simulink model "nn_fuel_control_4_20_1"  (R2021a)
settings: Solver=ode15s  StartTime=0.0  StopTime=T  MaxStep=.01  RelTol=1e-3
undefined symbols (not defined in the file): AF_sensor_tol, fault_time, fuel_inj_tol, kappa_tol, MAF_sensor_tol, pump_tol, tau_ww_tol
libraries: neural x86
(part 2 of 4)

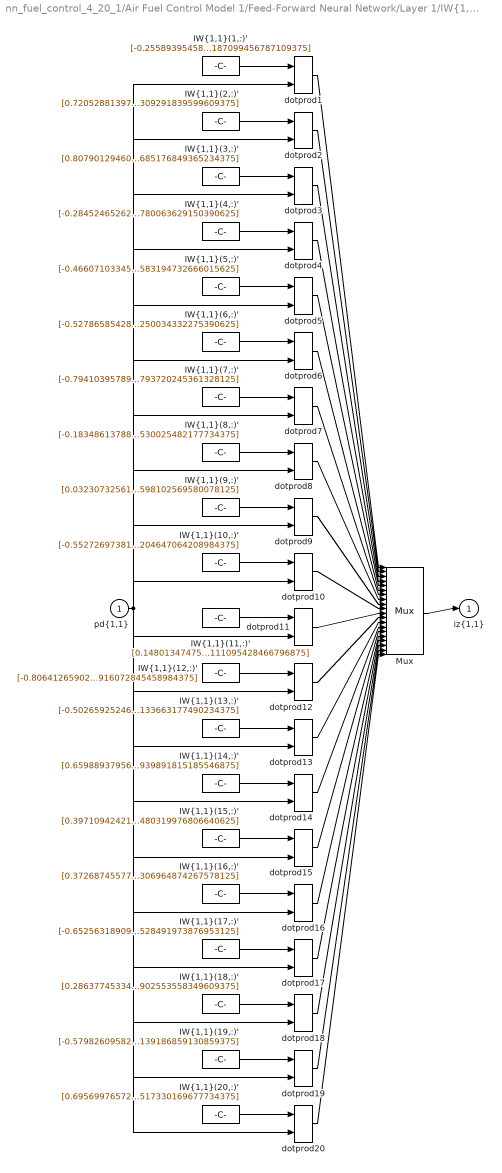
== system nn_fuel_control_4_20_1/Air Fuel Control Model 1/Feed-Forward Neural Network/Layer 1/IW{1,1} ==
  "pd{1,1}" : Inport  PortDimensions=4
      mask Display: e = 0.06;c1 = [120 230 180]/255;c2 = ([120 230 180]+0)/(256+128);c3 = ([120 230 180]+128)/(256+128);patch([0 1 1 0],[0 0 1 1],c1);patch([0 1 1 1-e 1-e 0+e],[0 0 1 1-e 0+e 0+e],c2);patch([0 0 1 1-e 0+e 0+e],[0 1 1 1-e 1-e 0+e],c3);plot([0 1 1 0 0],[0 0 1 1 0]);
  "IW{1,1}(1,:)'" : Constant  Value=[-0.255893954581917271173807648665388114750385284423828125;-0.050180613703053662810749102618501638062298297882080078125;-0.411204029772260393205129958005272783339023590087890625;-0.05416988303420254557973834153017378412187099456787109375]
      mask Display: e = 0.06;c1 = [120 150 230]/255;c2 = ([120 150 230]+0)/383;c3 = ([120 150 230]+128)/383;patch([0 1 1 0],[0 0 1 1],c1);patch([0 1 1 1-e 1-e 0+e],[0 0 1 1-e 0+e 0+e],c2);patch([0 0 1 1-e 0+e 0+e],[0 1 1 1-e 1-e 0+e],c3);plot([0 1 1 0 0],[0 0 1 1 0]);disp('Weights');
  "IW{1,1}(10,:)'" : Constant  Value=[-0.55272697381055768683921769479638896882534027099609375;-0.651499269241095912974515158566646277904510498046875;0.63947614252412832147598464871407486498355865478515625;-0.590736262891938590513518647640012204647064208984375]
      mask Display: e = 0.06;c1 = [120 150 230]/255;c2 = ([120 150 230]+0)/383;c3 = ([120 150 230]+128)/383;patch([0 1 1 0],[0 0 1 1],c1);patch([0 1 1 1-e 1-e 0+e],[0 0 1 1-e 0+e 0+e],c2);patch([0 0 1 1-e 0+e 0+e],[0 1 1 1-e 1-e 0+e],c3);plot([0 1 1 0 0],[0 0 1 1 0]);disp('Weights');
  "IW{1,1}(11,:)'" : Constant  Value=[0.1480134747547011409007922111413790844380855560302734375;0.6684648726112827343825983916758559644222259521484375;0.062198838454765502381516029117847210727632045745849609375;-0.60427407435323476914135198967414908111095428466796875]
      mask Display: e = 0.06;c1 = [120 150 230]/255;c2 = ([120 150 230]+0)/383;c3 = ([120 150 230]+128)/383;patch([0 1 1 0],[0 0 1 1],c1);patch([0 1 1 1-e 1-e 0+e],[0 0 1 1-e 0+e 0+e],c2);patch([0 0 1 1-e 0+e 0+e],[0 1 1 1-e 1-e 0+e],c3);plot([0 1 1 0 0],[0 0 1 1 0]);disp('Weights');
  "IW{1,1}(12,:)'" : Constant  Value=[-0.8064126590285745077579804274137131869792938232421875;-0.1946243266823513007324208956561051309108734130859375;0.05077726277785125919006503636410343460738658905029296875;0.71413696176898555645351507337181828916072845458984375]
      mask Display: e = 0.06;c1 = [120 150 230]/255;c2 = ([120 150 230]+0)/383;c3 = ([120 150 230]+128)/383;patch([0 1 1 0],[0 0 1 1],c1);patch([0 1 1 1-e 1-e 0+e],[0 0 1 1-e 0+e 0+e],c2);patch([0 0 1 1-e 0+e 0+e],[0 1 1 1-e 1-e 0+e],c3);plot([0 1 1 0 0],[0 0 1 1 0]);disp('Weights');
  "IW{1,1}(13,:)'" : Constant  Value=[-0.5026592524653068494444596581161022186279296875;-0.8442232439786565567629850193043239414691925048828125;-0.4600549917996483717530509238713420927524566650390625;-0.538643370776307417457928750081919133663177490234375]
      mask Display: e = 0.06;c1 = [120 150 230]/255;c2 = ([120 150 230]+0)/383;c3 = ([120 150 230]+128)/383;patch([0 1 1 0],[0 0 1 1],c1);patch([0 1 1 1-e 1-e 0+e],[0 0 1 1-e 0+e 0+e],c2);patch([0 0 1 1-e 0+e 0+e],[0 1 1 1-e 1-e 0+e],c3);plot([0 1 1 0 0],[0 0 1 1 0]);disp('Weights');
  "IW{1,1}(14,:)'" : Constant  Value=[0.6598893795696885167245682168868370354175567626953125;-0.66306349623711835494788147116196341812610626220703125;-0.016209493408949893211712378615629859268665313720703125;0.7971581335749486907360505938413552939891815185546875]
      mask Display: e = 0.06;c1 = [120 150 230]/255;c2 = ([120 150 230]+0)/383;c3 = ([120 150 230]+128)/383;patch([0 1 1 0],[0 0 1 1],c1);patch([0 1 1 1-e 1-e 0+e],[0 0 1 1-e 0+e 0+e],c2);patch([0 0 1 1-e 0+e 0+e],[0 1 1 1-e 1-e 0+e],c3);plot([0 1 1 0 0],[0 0 1 1 0]);disp('Weights');
  "IW{1,1}(15,:)'" : Constant  Value=[0.397109424219522555432604349334724247455596923828125;-0.97950665478874388014673968427814543247222900390625;-0.532533438767095912425020287628285586833953857421875;0.594249136505285324716396644362248480319976806640625]
      mask Display: e = 0.06;c1 = [120 150 230]/255;c2 = ([120 150 230]+0)/383;c3 = ([120 150 230]+128)/383;patch([0 1 1 0],[0 0 1 1],c1);patch([0 1 1 1-e 1-e 0+e],[0 0 1 1-e 0+e 0+e],c2);patch([0 0 1 1-e 0+e 0+e],[0 1 1 1-e 1-e 0+e],c3);plot([0 1 1 0 0],[0 0 1 1 0]);disp('Weights');
  "IW{1,1}(16,:)'" : Constant  Value=[0.372687455772187814506679615078610368072986602783203125;-0.90807611825004019845408720357227139174938201904296875;-0.457367237946180560381748136933310888707637786865234375;0.55645598307857035980106275019352324306964874267578125]
      mask Display: e = 0.06;c1 = [120 150 230]/255;c2 = ([120 150 230]+0)/383;c3 = ([120 150 230]+128)/383;patch([0 1 1 0],[0 0 1 1],c1);patch([0 1 1 1-e 1-e 0+e],[0 0 1 1-e 0+e 0+e],c2);patch([0 0 1 1-e 0+e 0+e],[0 1 1 1-e 1-e 0+e],c3);plot([0 1 1 0 0],[0 0 1 1 0]);disp('Weights');
  "IW{1,1}(17,:)'" : Constant  Value=[-0.6525631890917888977554639495792798697948455810546875;0.30110178388549169170573804876767098903656005859375;0.1303703819094477467377402035708655603229999542236328125;0.897007452078188993738194767502136528491973876953125]
      mask Display: e = 0.06;c1 = [120 150 230]/255;c2 = ([120 150 230]+0)/383;c3 = ([120 150 230]+128)/383;patch([0 1 1 0],[0 0 1 1],c1);patch([0 1 1 1-e 1-e 0+e],[0 0 1 1-e 0+e 0+e],c2);patch([0 0 1 1-e 0+e 0+e],[0 1 1 1-e 1-e 0+e],c3);plot([0 1 1 0 0],[0 0 1 1 0]);disp('Weights');
  "IW{1,1}(18,:)'" : Constant  Value=[0.286377453348653665532452805564389564096927642822265625;0.50923809025101751668529459493583999574184417724609375;-0.1177085687787508827550908563353004865348339080810546875;0.214421817752911803012239033705554902553558349609375]
      mask Display: e = 0.06;c1 = [120 150 230]/255;c2 = ([120 150 230]+0)/383;c3 = ([120 150 230]+128)/383;patch([0 1 1 0],[0 0 1 1],c1);patch([0 1 1 1-e 1-e 0+e],[0 0 1 1-e 0+e 0+e],c2);patch([0 0 1 1-e 0+e 0+e],[0 1 1 1-e 1-e 0+e],c3);plot([0 1 1 0 0],[0 0 1 1 0]);disp('Weights');
  "IW{1,1}(19,:)'" : Constant  Value=[-0.57982609582202027098674079752527177333831787109375;-0.563291776334291949268617827328853309154510498046875;0.100587291224137675982319706236012279987335205078125;0.1910173290938883550182936232886277139186859130859375]
      mask Display: e = 0.06;c1 = [120 150 230]/255;c2 = ([120 150 230]+0)/383;c3 = ([120 150 230]+128)/383;patch([0 1 1 0],[0 0 1 1],c1);patch([0 1 1 1-e 1-e 0+e],[0 0 1 1-e 0+e 0+e],c2);patch([0 0 1 1-e 0+e 0+e],[0 1 1 1-e 1-e 0+e],c3);plot([0 1 1 0 0],[0 0 1 1 0]);disp('Weights');
  "IW{1,1}(2,:)'" : Constant  Value=[0.72052881397894197323950038480688817799091339111328125;-0.1079570095728306367011128941157949157059192657470703125;0.280125365935717851595398997233132831752300262451171875;-0.31323344257810281643372718463069759309291839599609375]
      mask Display: e = 0.06;c1 = [120 150 230]/255;c2 = ([120 150 230]+0)/383;c3 = ([120 150 230]+128)/383;patch([0 1 1 0],[0 0 1 1],c1);patch([0 1 1 1-e 1-e 0+e],[0 0 1 1-e 0+e 0+e],c2);patch([0 0 1 1-e 0+e 0+e],[0 1 1 1-e 1-e 0+e],c3);plot([0 1 1 0 0],[0 0 1 1 0]);disp('Weights');
  "IW{1,1}(20,:)'" : Constant  Value=[0.69569976572952452187337257782928645610809326171875;-0.158886500019682130879772330445121042430400848388671875;1.0467247081747499404258405775181017816066741943359375;-0.786786319988487914400820955052040517330169677734375]
      mask Display: e = 0.06;c1 = [120 150 230]/255;c2 = ([120 150 230]+0)/383;c3 = ([120 150 230]+128)/383;patch([0 1 1 0],[0 0 1 1],c1);patch([0 1 1 1-e 1-e 0+e],[0 0 1 1-e 0+e 0+e],c2);patch([0 0 1 1-e 0+e 0+e],[0 1 1 1-e 1-e 0+e],c3);plot([0 1 1 0 0],[0 0 1 1 0]);disp('Weights');
  "IW{1,1}(3,:)'" : Constant  Value=[0.80790129460351567391995786238112486898899078369140625;0.60020113472108682639571952677215449512004852294921875;-0.743655296177256008860467773047275841236114501953125;-0.1015119663675712879946644306983216665685176849365234375]
      mask Display: e = 0.06;c1 = [120 150 230]/255;c2 = ([120 150 230]+0)/383;c3 = ([120 150 230]+128)/383;patch([0 1 1 0],[0 0 1 1],c1);patch([0 1 1 1-e 1-e 0+e],[0 0 1 1-e 0+e 0+e],c2);patch([0 0 1 1-e 0+e 0+e],[0 1 1 1-e 1-e 0+e],c3);plot([0 1 1 0 0],[0 0 1 1 0]);disp('Weights');
  "IW{1,1}(4,:)'" : Constant  Value=[-0.28452465262175674620692689131828956305980682373046875;-0.1455400286438181256531976259793736971914768218994140625;0.2090543561159994012665919171922723762691020965576171875;0.3143679152500846729623162900679744780063629150390625]
      mask Display: e = 0.06;c1 = [120 150 230]/255;c2 = ([120 150 230]+0)/383;c3 = ([120 150 230]+128)/383;patch([0 1 1 0],[0 0 1 1],c1);patch([0 1 1 1-e 1-e 0+e],[0 0 1 1-e 0+e 0+e],c2);patch([0 0 1 1-e 0+e 0+e],[0 1 1 1-e 1-e 0+e],c3);plot([0 1 1 0 0],[0 0 1 1 0]);disp('Weights');
  "IW{1,1}(5,:)'" : Constant  Value=[-0.46607103345306055697250258162966929376125335693359375;0.4045752847885430991681232626433484256267547607421875;-0.2487346108752874485059436437950353138148784637451171875;-0.8540124870413221547238435960025526583194732666015625]
      mask Display: e = 0.06;c1 = [120 150 230]/255;c2 = ([120 150 230]+0)/383;c3 = ([120 150 230]+128)/383;patch([0 1 1 0],[0 0 1 1],c1);patch([0 1 1 1-e 1-e 0+e],[0 0 1 1-e 0+e 0+e],c2);patch([0 0 1 1-e 0+e 0+e],[0 1 1 1-e 1-e 0+e],c3);plot([0 1 1 0 0],[0 0 1 1 0]);disp('Weights');
  "IW{1,1}(6,:)'" : Constant  Value=[-0.52786585428759724702985067779081873595714569091796875;0.56258148622816828154924451155238784849643707275390625;0.1597122724516217562307218713613110594451427459716796875;-0.56017202948027000619646287304931320250034332275390625]
      mask Display: e = 0.06;c1 = [120 150 230]/255;c2 = ([120 150 230]+0)/383;c3 = ([120 150 230]+128)/383;patch([0 1 1 0],[0 0 1 1],c1);patch([0 1 1 1-e 1-e 0+e],[0 0 1 1-e 0+e 0+e],c2);patch([0 0 1 1-e 0+e 0+e],[0 1 1 1-e 1-e 0+e],c3);plot([0 1 1 0 0],[0 0 1 1 0]);disp('Weights');
  "IW{1,1}(7,:)'" : Constant  Value=[-0.7941039578996564873847319177002646028995513916015625;0.402454842875472562635508211315027438104152679443359375;-1.1760264490640590651082675321958959102630615234375;0.4049690339423961393805484476615674793720245361328125]
      mask Display: e = 0.06;c1 = [120 150 230]/255;c2 = ([120 150 230]+0)/383;c3 = ([120 150 230]+128)/383;patch([0 1 1 0],[0 0 1 1],c1);patch([0 1 1 1-e 1-e 0+e],[0 0 1 1-e 0+e 0+e],c2);patch([0 0 1 1-e 0+e 0+e],[0 1 1 1-e 1-e 0+e],c3);plot([0 1 1 0 0],[0 0 1 1 0]);disp('Weights');
  "IW{1,1}(8,:)'" : Constant  Value=[-0.1834861378839762746650876579224132001399993896484375;-0.2696005694128247309748758198111318051815032958984375;0.0449899432481253302995582998846657574176788330078125;0.40879506644844099128022207878530025482177734375]
      mask Display: e = 0.06;c1 = [120 150 230]/255;c2 = ([120 150 230]+0)/383;c3 = ([120 150 230]+128)/383;patch([0 1 1 0],[0 0 1 1],c1);patch([0 1 1 1-e 1-e 0+e],[0 0 1 1-e 0+e 0+e],c2);patch([0 0 1 1-e 0+e 0+e],[0 1 1 1-e 1-e 0+e],c3);plot([0 1 1 0 0],[0 0 1 1 0]);disp('Weights');
  "IW{1,1}(9,:)'" : Constant  Value=[0.0323073256130863573076794637017883360385894775390625;0.3668530899902517905530885400366969406604766845703125;-0.620161838295766099093953016563318669795989990234375;-0.9815621933458509307257600084994919598102569580078125]
      mask Display: e = 0.06;c1 = [120 150 230]/255;c2 = ([120 150 230]+0)/383;c3 = ([120 150 230]+128)/383;patch([0 1 1 0],[0 0 1 1],c1);patch([0 1 1 1-e 1-e 0+e],[0 0 1 1-e 0+e 0+e],c2);patch([0 0 1 1-e 0+e 0+e],[0 1 1 1-e 1-e 0+e],c3);plot([0 1 1 0 0],[0 0 1 1 0]);disp('Weights');
  Mux : Mux  Inputs=20
      mask Display: e = 0.06;c1 = [120 150 230]/255;c2 = ([120 150 230]+0)/383;c3 = ([120 150 230]+128)/383;patch([0 1 1 0],[0 0 1 1],c1);patch([0 1 1 1-e 1-e 0+e],[0 0 1 1-e 0+e 0+e],c2);patch([0 0 1 1-e 0+e 0+e],[0 1 1 1-e 1-e 0+e],c3);plot([0 1 1 0 0],[0 0 1 1 0]);disp('Mux');
  dotprod{1..20} (20 alike) : neural/Weight Functions/dotprod
  "iz{1,1}" : Outport
      mask Display: e = 0.06;c1 = [120 230 180]/255;c2 = ([120 230 180]+0)/(256+128);c3 = ([120 230 180]+128)/(256+128);patch([0 1 1 0],[0 0 1 1],c1);patch([0 1 1 1-e 1-e 0+e],[0 0 1 1-e 0+e 0+e],c2);patch([0 0 1 1-e 0+e 0+e],[0 1 1 1-e 1-e 0+e],c3);plot([0 1 1 0 0],[0 0 1 1 0]);
  wires:
  "IW{1,1}(1,:)'"/1 -> dotprod1/1
  "pd{1,1}"/1 -> dotprod1/2, dotprod2/2, dotprod3/2, dotprod4/2, dotprod5/2, dotprod6/2, dotprod7/2, dotprod8/2, dotprod9/2, dotprod10/2, dotprod11/2, dotprod12/2, dotprod13/2, dotprod14/2, dotprod15/2, dotprod16/2, dotprod17/2, dotprod18/2, dotprod19/2, dotprod20/2
  dotprod1/1 -> Mux/1
  "IW{1,1}(2,:)'"/1 -> dotprod2/1
  dotprod2/1 -> Mux/2
  "IW{1,1}(3,:)'"/1 -> dotprod3/1
  dotprod3/1 -> Mux/3
  "IW{1,1}(4,:)'"/1 -> dotprod4/1
  dotprod4/1 -> Mux/4
  "IW{1,1}(5,:)'"/1 -> dotprod5/1
  dotprod5/1 -> Mux/5
  "IW{1,1}(6,:)'"/1 -> dotprod6/1
  dotprod6/1 -> Mux/6
  "IW{1,1}(7,:)'"/1 -> dotprod7/1
  dotprod7/1 -> Mux/7
  "IW{1,1}(8,:)'"/1 -> dotprod8/1
  dotprod8/1 -> Mux/8
  "IW{1,1}(9,:)'"/1 -> dotprod9/1
  dotprod9/1 -> Mux/9
  "IW{1,1}(10,:)'"/1 -> dotprod10/1
  dotprod10/1 -> Mux/10
  "IW{1,1}(11,:)'"/1 -> dotprod11/1
  dotprod11/1 -> Mux/11
  "IW{1,1}(12,:)'"/1 -> dotprod12/1
  dotprod12/1 -> Mux/12
  "IW{1,1}(13,:)'"/1 -> dotprod13/1
  dotprod13/1 -> Mux/13
  "IW{1,1}(14,:)'"/1 -> dotprod14/1
  dotprod14/1 -> Mux/14
  "IW{1,1}(15,:)'"/1 -> dotprod15/1
  dotprod15/1 -> Mux/15
  "IW{1,1}(16,:)'"/1 -> dotprod16/1
  dotprod16/1 -> Mux/16
  "IW{1,1}(17,:)'"/1 -> dotprod17/1
  dotprod17/1 -> Mux/17
  "IW{1,1}(18,:)'"/1 -> dotprod18/1
  dotprod18/1 -> Mux/18
  "IW{1,1}(19,:)'"/1 -> dotprod19/1
  dotprod19/1 -> Mux/19
  "IW{1,1}(20,:)'"/1 -> dotprod20/1
  dotprod20/1 -> Mux/20
  Mux/1 -> "iz{1,1}"/1

== system nn_fuel_control_4_20_1/Air Fuel Control Model 1/Feed-Forward Neural Network/Layer 2/Delays 1 ==
  "p{2}" : Inport  PortDimensions=20
      mask Display: e = 0.06;c1 = [120 230 180]/255;c2 = ([120 230 180]+0)/(256+128);c3 = ([120 230 180]+128)/(256+128);patch([0 1 1 0],[0 0 1 1],c1);patch([0 1 1 1-e 1-e 0+e],[0 0 1 1-e 0+e 0+e],c2);patch([0 0 1 1-e 0+e 0+e],[0 1 1 1-e 1-e 0+e],c3);plot([0 1 1 0 0],[0 0 1 1 0]);
  mux : Mux  Inputs=1
      mask Display: e = 0.06;c1 = [120 150 230]/255;c2 = ([120 150 230]+0)/383;c3 = ([120 150 230]+128)/383;patch([0 1 1 0],[0 0 1 1],c1);patch([0 1 1 1-e 1-e 0+e],[0 0 1 1-e 0+e 0+e],c2);patch([0 0 1 1-e 0+e 0+e],[0 1 1 1-e 1-e 0+e],c3);plot([0 1 1 0 0],[0 0 1 1 0]);disp('Mux')
  "pd{2,1}" : Outport
      mask Display: e = 0.06;c1 = [120 230 180]/255;c2 = ([120 230 180]+0)/(256+128);c3 = ([120 230 180]+128)/(256+128);patch([0 1 1 0],[0 0 1 1],c1);patch([0 1 1 1-e 1-e 0+e],[0 0 1 1-e 0+e 0+e],c2);patch([0 0 1 1-e 0+e 0+e],[0 1 1 1-e 1-e 0+e],c3);plot([0 1 1 0 0],[0 0 1 1 0]);
  wires:
  "p{2}"/1 -> mux/1
  mux/1 -> "pd{2,1}"/1

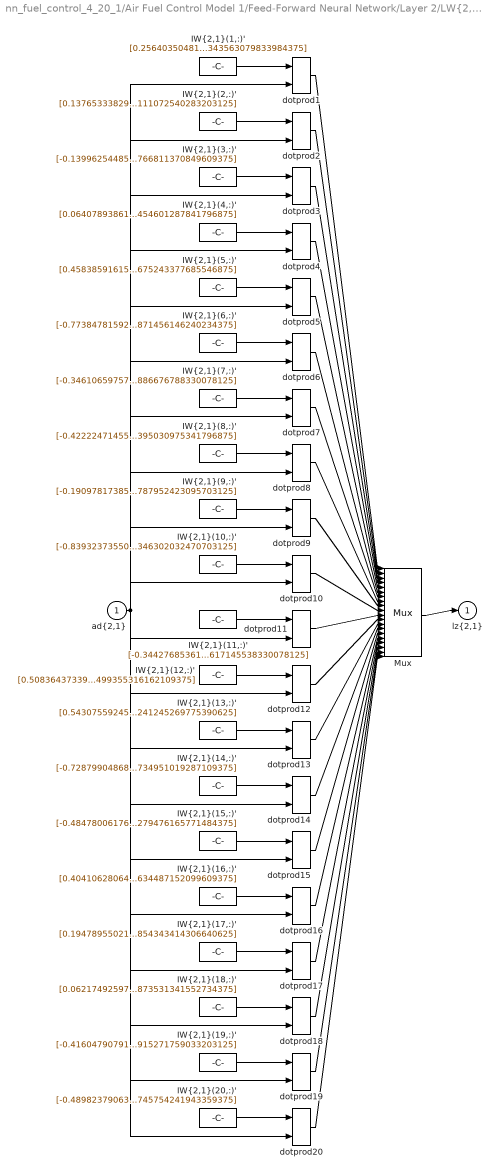
== system nn_fuel_control_4_20_1/Air Fuel Control Model 1/Feed-Forward Neural Network/Layer 2/LW{2,1} ==
  "ad{2,1}" : Inport  PortDimensions=20
      mask Display: e = 0.06;c1 = [120 230 180]/255;c2 = ([120 230 180]+0)/(256+128);c3 = ([120 230 180]+128)/(256+128);patch([0 1 1 0],[0 0 1 1],c1);patch([0 1 1 1-e 1-e 0+e],[0 0 1 1-e 0+e 0+e],c2);patch([0 0 1 1-e 0+e 0+e],[0 1 1 1-e 1-e 0+e],c3);plot([0 1 1 0 0],[0 0 1 1 0]);
  "IW{2,1}(1,:)'" : Constant  Value=[0.256403504819027683314658361268811859190464019775390625;0.55699273716688690871734479514998383820056915283203125;-0.10243484263037373749316572002499015070497989654541015625;0.61017359243633340071255588554777204990386962890625;-0.49168853908283549625224395640543662011623382568359375;-0.445185796413017254025135116535238921642303466796875;0.66658292791435036495073518381104804575443267822265625;0.74941831651127532865075409063138067722320556640625;0.348045444215012711453027804964222013950347900390625;0.86509340571704573807920723993447609245777130126953125;0.74428775142764858063770816443138755857944488525390625;-0.6684261822986099499388501499197445809841156005859375;0.821552287158203053962779449648223817348480224609375;0.06921567489521453231393621763345436193048954010009765625;0.69405408543870894533256432623602449893951416015625;-0.08884209416376896706335486442185356281697750091552734375;0.1065002363070592095173338975655497051775455474853515625;0.9502109393119704261465585659607313573360443115234375;0.3213179247461728227364119447884149849414825439453125;-0.48618430376372800960638187461881898343563079833984375]
      mask Display: e = 0.06;c1 = [120 150 230]/255;c2 = ([120 150 230]+0)/383;c3 = ([120 150 230]+128)/383;patch([0 1 1 0],[0 0 1 1],c1);patch([0 1 1 1-e 1-e 0+e],[0 0 1 1-e 0+e 0+e],c2);patch([0 0 1 1-e 0+e 0+e],[0 1 1 1-e 1-e 0+e],c3);plot([0 1 1 0 0],[0 0 1 1 0]);disp('weights');
  "IW{2,1}(10,:)'" : Constant  Value=[-0.839323735500342227311421083868481218814849853515625;-0.1027802378071994426900204189223586581647396087646484375;-0.7806964202693096321894472566782496869564056396484375;0.680681515772560086219300501397810876369476318359375;-0.51100504457678008751742027016007341444492340087890625;-0.51150485750802621165433947680867277085781097412109375;-0.1924599703979477938187159224980860017240047454833984375;-0.3642331759206876018453158394549973309040069580078125;0.4202409374541262732094537568627856671810150146484375;-0.64692134435889148136311632697470486164093017578125;-0.49688718155034805601388825380126945674419403076171875;0.5581295053278108042604799265973269939422607421875;-0.4857655414840549301658256808877922594547271728515625;-0.41702184565919953040946666078525595366954803466796875;-0.3202437589281850183198230297421105206012725830078125;-0.9406677162011334303315379656851291656494140625;0.7897233817597302252266899813548661768436431884765625;-0.70530703875142897185668289239401929080486297607421875;-0.197104048309090007506938491133041679859161376953125;-0.9954045937389335296785475293290801346302032470703125]
      mask Display: e = 0.06;c1 = [120 150 230]/255;c2 = ([120 150 230]+0)/383;c3 = ([120 150 230]+128)/383;patch([0 1 1 0],[0 0 1 1],c1);patch([0 1 1 1-e 1-e 0+e],[0 0 1 1-e 0+e 0+e],c2);patch([0 0 1 1-e 0+e 0+e],[0 1 1 1-e 1-e 0+e],c3);plot([0 1 1 0 0],[0 0 1 1 0]);disp('weights');
  "IW{2,1}(11,:)'" : Constant  Value=[-0.3442768536160334402751459492719732224941253662109375;-0.126645193186832150100684657445526681840419769287109375;-0.25582239816656604514122363980277441442012786865234375;-0.475188837819449261257176431172410957515239715576171875;-0.380699988172073233716474760512937791645526885986328125;0.6681082596167755571769930611480958759784698486328125;0.61680611870214019365477042811107821762561798095703125;-0.3842982728840949047111053005210123956203460693359375;0.092199959895641558915713176247663795948028564453125;0.646735751844751849404246968333609402179718017578125;-0.3566726201985510602554541037534363567829132080078125;0.862487777138273514765387517400085926055908203125;0.3401193911093225441533149933093227446079254150390625;-0.88438663542802509187623627440189011394977569580078125;-0.2883601808382836306776653145789168775081634521484375;1.13845020905304039615657529793679714202880859375;-0.98259045851291926254589270683936774730682373046875;0.3131654024901433519545435046893544495105743408203125;-0.40667411652741325411852812976576387882232666015625;0.88431093975587338196220343888853676617145538330078125]
      mask Display: e = 0.06;c1 = [120 150 230]/255;c2 = ([120 150 230]+0)/383;c3 = ([120 150 230]+128)/383;patch([0 1 1 0],[0 0 1 1],c1);patch([0 1 1 1-e 1-e 0+e],[0 0 1 1-e 0+e 0+e],c2);patch([0 0 1 1-e 0+e 0+e],[0 1 1 1-e 1-e 0+e],c3);plot([0 1 1 0 0],[0 0 1 1 0]);disp('weights');
  "IW{2,1}(12,:)'" : Constant  Value=[0.5083643733909475326271376616205088794231414794921875;0.6979322964989373989652676755213178694248199462890625;0.92178415717860884281975586418411694467067718505859375;-0.39033104832621534630021642442443408071994781494140625;-0.383678218211015054084356279417988844215869903564453125;-0.61391769395999717939815809586434625089168548583984375;-0.591094668264378952926563215442001819610595703125;-0.312979327589984368529485436738468706607818603515625;-0.0842029111634989835266651425627060234546661376953125;-0.8006509914526864779560355600551702082157135009765625;-0.10037107631365442539372878627546015195548534393310546875;0.551034974300382174305923399515450000762939453125;0.7040581567920323191600573409232310950756072998046875;0.059419260238086461789475123396186972968280315399169921875;0.483832787080651360867022958700545132160186767578125;-0.6947366657908133902310510165989398956298828125;0.188227171095658951660567481667385436594486236572265625;-0.24625857672740936177291359854280017316341400146484375;0.0379784065678607785088161108433268964290618896484375;-0.1936138778400245674671253937049186788499355316162109375]
      mask Display: e = 0.06;c1 = [120 150 230]/255;c2 = ([120 150 230]+0)/383;c3 = ([120 150 230]+128)/383;patch([0 1 1 0],[0 0 1 1],c1);patch([0 1 1 1-e 1-e 0+e],[0 0 1 1-e 0+e 0+e],c2);patch([0 0 1 1-e 0+e 0+e],[0 1 1 1-e 1-e 0+e],c3);plot([0 1 1 0 0],[0 0 1 1 0]);disp('weights');
  "IW{2,1}(13,:)'" : Constant  Value=[0.54307559245790348878557551870471797883510589599609375;0.75271368477932398821650394893367774784564971923828125;-0.1275235670257674203131870172001072205603122711181640625;-0.58684458116446325259829563947278074920177459716796875;0.9795271839011350234471819931059144437313079833984375;0.115565273299358672876024911602144129574298858642578125;0.11335394344267306354634428089411812834441661834716796875;0.358539371416803920311622277949936687946319580078125;-0.0126515875916339837203850038349628448486328125;-0.260894828747942231217393782571889460086822509765625;0.1574081397651138358728672983488650061190128326416015625;0.1420118999546165217129356506120529957115650177001953125;0.5099030275380067589452437459840439260005950927734375;-0.81828653190900879632607711755554191768169403076171875;-0.1545897804274993792006398507510311901569366455078125;0.675439808810708530728561527212150394916534423828125;-0.127791243383908181829866634870995767414569854736328125;0.98852637578982560651041922028525732457637786865234375;0.0986064542185760561920915279188193380832672119140625;0.01154229721346903582424037182363463216461241245269775390625]
      mask Display: e = 0.06;c1 = [120 150 230]/255;c2 = ([120 150 230]+0)/383;c3 = ([120 150 230]+128)/383;patch([0 1 1 0],[0 0 1 1],c1);patch([0 1 1 1-e 1-e 0+e],[0 0 1 1-e 0+e 0+e],c2);patch([0 0 1 1-e 0+e 0+e],[0 1 1 1-e 1-e 0+e],c3);plot([0 1 1 0 0],[0 0 1 1 0]);disp('weights');
  "IW{2,1}(14,:)'" : Constant  Value=[-0.728799048689657613664394375518895685672760009765625;-0.296529345416541800783960525222937576472759246826171875;-0.7972119443543326244849822614924050867557525634765625;-1.0118923326638957771450577638461254537105560302734375;-0.5272267009729585396371476235799491405487060546875;-0.8855868557823221021152448884095065295696258544921875;0.5121663467363941624199696889263577759265899658203125;0.2545828879630407381995382820605300366878509521484375;0.6292814383810225731252785408287309110164642333984375;-0.929475350504611608215554952039383351802825927734375;0.069808995965472020461817237446666695177555084228515625;0.7352931823411916756327855182462371885776519775390625;-0.7827631248789221896089429719722829759120941162109375;-0.537355068723539108788145313155837357044219970703125;0.4990633751586894817364736809395253658294677734375;0.10586567362169052586295947548933327198028564453125;0.7861825800106121420185445458628237247467041015625;-0.8456802487706689408497595650260336697101593017578125;-0.015314959104377745546798905706964433193206787109375;-0.2971057125480276450701921930885873734951019287109375]
      mask Display: e = 0.06;c1 = [120 150 230]/255;c2 = ([120 150 230]+0)/383;c3 = ([120 150 230]+128)/383;patch([0 1 1 0],[0 0 1 1],c1);patch([0 1 1 1-e 1-e 0+e],[0 0 1 1-e 0+e 0+e],c2);patch([0 0 1 1-e 0+e 0+e],[0 1 1 1-e 1-e 0+e],c3);plot([0 1 1 0 0],[0 0 1 1 0]);disp('weights');
  "IW{2,1}(15,:)'" : Constant  Value=[-0.484780061765159142606052000701311044394969940185546875;-0.415234292406290117494194191749556921422481536865234375;-1.0346574979893914392192755258292891085147857666015625;-0.402016275094312536264595792090403847396373748779296875;-0.138088078526567181736339762210263870656490325927734375;0.87346766333678382832061970475479029119014739990234375;0.441802139086038103688025557858054526150226593017578125;-0.1309872596360344143562315366580151021480560302734375;-0.610204389748495668044370177085511386394500732421875;-0.03839265832583131643485074846466886810958385467529296875;0.249243117002509839696955395993427373468875885009765625;0.11801074905021964600582151661001262255012989044189453125;-0.2659363890055583823368579032830893993377685546875;-0.71930459889416187291288906635600142180919647216796875;-0.075520266869505636719850372173823416233062744140625;0.06868026364486297385969493234370020218193531036376953125;-0.89298865365537405391904712814721278846263885498046875;-0.215387890558910999327935087421792559325695037841796875;-0.2384945521682781954808660884737037122249603271484375;-0.62116688404883591001492959549068473279476165771484375]
      mask Display: e = 0.06;c1 = [120 150 230]/255;c2 = ([120 150 230]+0)/383;c3 = ([120 150 230]+128)/383;patch([0 1 1 0],[0 0 1 1],c1);patch([0 1 1 1-e 1-e 0+e],[0 0 1 1-e 0+e 0+e],c2);patch([0 0 1 1-e 0+e 0+e],[0 1 1 1-e 1-e 0+e],c3);plot([0 1 1 0 0],[0 0 1 1 0]);disp('weights');
  "IW{2,1}(16,:)'" : Constant  Value=[0.404106280640281256832935241618542931973934173583984375;0.70242360718233898264628578544943593442440032958984375;0.1641145711031210263630697454573237337172031402587890625;-0.247221087020352836560732612269930541515350341796875;0.05562678511628217636886262198459007777273654937744140625;-0.0072461926376732911647682300326778204180300235748291015625;0.1324024557175408622899936972316936589777469635009765625;-0.92978342018724191575529403053224086761474609375;0.56556497776320835413343957043252885341644287109375;0.3397230627633225363837254917598329484462738037109375;0.29431922470979732242568616129574365913867950439453125;0.51626009844002884729974311994737945497035980224609375;-0.6489613631160897622152106123394332826137542724609375;-0.24239263777640218666675764325191266834735870361328125;-0.5586844817010707675564162855152972042560577392578125;0.0290138265195338147794945626856133458204567432403564453125;0.6115143731481691435902803277713246643543243408203125;0.1748207830102221638224335720224189572036266326904296875;0.4941049018132852577167568597360514104366302490234375;0.33386371882758003604152463594800792634487152099609375]
      mask Display: e = 0.06;c1 = [120 150 230]/255;c2 = ([120 150 230]+0)/383;c3 = ([120 150 230]+128)/383;patch([0 1 1 0],[0 0 1 1],c1);patch([0 1 1 1-e 1-e 0+e],[0 0 1 1-e 0+e 0+e],c2);patch([0 0 1 1-e 0+e 0+e],[0 1 1 1-e 1-e 0+e],c3);plot([0 1 1 0 0],[0 0 1 1 0]);disp('weights');
  "IW{2,1}(17,:)'" : Constant  Value=[0.1947895502174626092273257427223143167793750762939453125;-0.52361898938939310799156601206050254404544830322265625;-0.10622093506646522464986759359817369841039180755615234375;-0.7466049808737535986580269309342838823795318603515625;0.427384088335486078680247601369046606123447418212890625;1.4693398718208683373376288727740757167339324951171875;-1.3104810676142888414830167675972916185855865478515625;0.4855049744317463389364775139256380498409271240234375;0.88199212165116680495202672318555414676666259765625;-0.60955399776535756917184016856481321156024932861328125;-0.54285148849283759719952513478347100317478179931640625;-0.70516678840002133821229790555662475526332855224609375;-0.41511492758453183427036492503248155117034912109375;0.6704157094871272537517370437853969633579254150390625;0.839123341803627909030183218419551849365234375;0.63222268412543380922130609178566373884677886962890625;-0.50732264518261949159949608656461350619792938232421875;-0.74154304207597621090286565959104336798191070556640625;-0.8111671411077410187573377697844989597797393798828125;-0.428285368422044288028160963222035206854343414306640625]
      mask Display: e = 0.06;c1 = [120 150 230]/255;c2 = ([120 150 230]+0)/383;c3 = ([120 150 230]+128)/383;patch([0 1 1 0],[0 0 1 1],c1);patch([0 1 1 1-e 1-e 0+e],[0 0 1 1-e 0+e 0+e],c2);patch([0 0 1 1-e 0+e 0+e],[0 1 1 1-e 1-e 0+e],c3);plot([0 1 1 0 0],[0 0 1 1 0]);disp('weights');
  "IW{2,1}(18,:)'" : Constant  Value=[0.06217492597023745182216458715629414655268192291259765625;-0.81824560730074236136744048053515143692493438720703125;-0.89641287430782690126562783916597254574298858642578125;-0.18391094474156732818670434426167048513889312744140625;0.9844616979050770932957448167144320905208587646484375;0.65484074414303805600212626814027316868305206298828125;-0.7925667457472191923528725965297780930995941162109375;0.0673400334330274130678617439116351306438446044921875;-0.083604201131516564515777645283378660678863525390625;0.58893929866951510998518415362923406064510345458984375;-0.94534449182464685978999341386952437460422515869140625;0.457648829261737388751640764894546009600162506103515625;0.1025857773266978245629843513597734272480010986328125;0.54381759553698583165015634222072549164295196533203125;0.5443058289233437818666061502881348133087158203125;-1.036147741921205511772541285608895123004913330078125;-0.24802282339544390321606215366045944392681121826171875;-0.9227639004882857154399289356661029160022735595703125;0.010338230956161709173102281056344509124755859375;-0.22463957916662502523053035474731586873531341552734375]
      mask Display: e = 0.06;c1 = [120 150 230]/255;c2 = ([120 150 230]+0)/383;c3 = ([120 150 230]+128)/383;patch([0 1 1 0],[0 0 1 1],c1);patch([0 1 1 1-e 1-e 0+e],[0 0 1 1-e 0+e 0+e],c2);patch([0 0 1 1-e 0+e 0+e],[0 1 1 1-e 1-e 0+e],c3);plot([0 1 1 0 0],[0 0 1 1 0]);disp('weights');
  "IW{2,1}(19,:)'" : Constant  Value=[-0.416047907917482195916392129220184870064258575439453125;0.309121326860066714115049535394064150750637054443359375;-0.0851180957864090814712909605077584274113178253173828125;0.339056785143795114123577150166966021060943603515625;-0.3096899454485384506341461019474081695079803466796875;-0.027548179279832142596351474139737547375261783599853515625;0.5216670052960143966203077070531435310840606689453125;-0.9988357428048779684814917345647700130939483642578125;-0.0344484434883864931720154345384798943996429443359375;-0.13242871890093044218161821845569647848606109619140625;0.522090219246575060196846607141196727752685546875;0.59382139028936331559549444136791862547397613525390625;-0.472735042050936637991753741516731679439544677734375;-0.74187595298605690796733824754483066499233245849609375;0.9082521364400701902042101210099644958972930908203125;0.551414488237109257084966884576715528964996337890625;0.2127486436982679307572396965042571537196636199951171875;0.91331207772785572007734344879281707108020782470703125;-0.8915657199296169732605221724952571094036102294921875;0.304700671032038183927426189256948418915271759033203125]
      mask Display: e = 0.06;c1 = [120 150 230]/255;c2 = ([120 150 230]+0)/383;c3 = ([120 150 230]+128)/383;patch([0 1 1 0],[0 0 1 1],c1);patch([0 1 1 1-e 1-e 0+e],[0 0 1 1-e 0+e 0+e],c2);patch([0 0 1 1-e 0+e 0+e],[0 1 1 1-e 1-e 0+e],c3);plot([0 1 1 0 0],[0 0 1 1 0]);disp('weights');
  "IW{2,1}(2,:)'" : Constant  Value=[0.137653338293227733846180171894957311451435089111328125;-0.460904548992435214582741309641278348863124847412109375;-0.290558282766146314113342441487475298345088958740234375;-0.63113207125823567178457551563042216002941131591796875;-0.517856009400533334741112412302754819393157958984375;-0.522612663993072157353481088648550212383270263671875;-1.14371085022362262151318645919673144817352294921875;-0.296969721859859259183167523588053882122039794921875;0.024219358823902581434595049358904361724853515625;0.247160225307312242382096201254171319305896759033203125;0.46439009629174032856013809578143991529941558837890625;0.053387629679267745164139569169492460787296295166015625;-0.1041289206064270889129375063930638134479522705078125;-0.00838366847669662351716368675624835304915904998779296875;-0.0691640104665527388760892790742218494415283203125;0.259218969043773894700422033565700985491275787353515625;0.197015094634830856268337129222345538437366485595703125;-0.171531257694670757896204804637818597257137298583984375;0.3180435006853030710516350154648534953594207763671875;0.00376749716591924521669199066309374757111072540283203125]
      mask Display: e = 0.06;c1 = [120 150 230]/255;c2 = ([120 150 230]+0)/383;c3 = ([120 150 230]+128)/383;patch([0 1 1 0],[0 0 1 1],c1);patch([0 1 1 1-e 1-e 0+e],[0 0 1 1-e 0+e 0+e],c2);patch([0 0 1 1-e 0+e 0+e],[0 1 1 1-e 1-e 0+e],c3);plot([0 1 1 0 0],[0 0 1 1 0]);disp('weights');
  "IW{2,1}(20,:)'" : Constant  Value=[-0.48982379063714720501820920617319643497467041015625;-0.1565414567378254073748422570133698172867298126220703125;1.0092678630572751163896327852853573858737945556640625;0.04997173210835093026815911798621527850627899169921875;-0.2079386696337817141966297640465199947357177734375;-0.321525828659411760934716539850342087447643280029296875;0.89409571631389106460829907518927939236164093017578125;0.5543458800608702663481608396978117525577545166015625;-0.49306510763555611021047297981567680835723876953125;0.27814303195336009810745281356503255665302276611328125;-0.81464293081563654563836962552159093320369720458984375;-0.35123732988197675641828254811116494238376617431640625;0.559540544336689205096035948372446000576019287109375;0.74652085046993865713460536426282487809658050537109375;0.28824650081486868913316357065923511981964111328125;-0.6182866746032604776672769730794243514537811279296875;-1.0877338496879047635701454055379144847393035888671875;-0.104371293272435661236841042409650981426239013671875;-0.913504009541565853425026944023557007312774658203125;-0.07584107192232168725976038103908649645745754241943359375]
      mask Display: e = 0.06;c1 = [120 150 230]/255;c2 = ([120 150 230]+0)/383;c3 = ([120 150 230]+128)/383;patch([0 1 1 0],[0 0 1 1],c1);patch([0 1 1 1-e 1-e 0+e],[0 0 1 1-e 0+e 0+e],c2);patch([0 0 1 1-e 0+e 0+e],[0 1 1 1-e 1-e 0+e],c3);plot([0 1 1 0 0],[0 0 1 1 0]);disp('weights');
  "IW{2,1}(3,:)'" : Constant  Value=[-0.13996254485875747608503161245607770979404449462890625;0.40060507371922027264332655249745585024356842041015625;-0.56815400850477704164376291373628191649913787841796875;-0.36553702608923399619555993922404013574123382568359375;-0.2482509998169468434792150901557761244475841522216796875;0.87407339206503975592710276032448746263980865478515625;0.893528192848337621256860074936412274837493896484375;0.632635861991303727336344309151172637939453125;0.869699939278778533235936265555210411548614501953125;0.98773112363063086949210855891578830778598785400390625;0.85399909375677662826120695171994157135486602783203125;-0.32594369818186275100657667280756868422031402587890625;0.4629603075816663970698527919012121856212615966796875;0.04308516642885058811618392837772262282669544219970703125;-0.231801523593062608341597297112457454204559326171875;-1.1623640803209145389018885907717049121856689453125;-0.88408872473551369797206689327140338718891143798828125;-0.8663309035618642628406860239920206367969512939453125;0.765185547700010459948316565714776515960693359375;-0.58307506602012215690677976454026065766811370849609375]
      mask Display: e = 0.06;c1 = [120 150 230]/255;c2 = ([120 150 230]+0)/383;c3 = ([120 150 230]+128)/383;patch([0 1 1 0],[0 0 1 1],c1);patch([0 1 1 1-e 1-e 0+e],[0 0 1 1-e 0+e 0+e],c2);patch([0 0 1 1-e 0+e 0+e],[0 1 1 1-e 1-e 0+e],c3);plot([0 1 1 0 0],[0 0 1 1 0]);disp('weights');
  "IW{2,1}(4,:)'" : Constant  Value=[0.064078938617030456459389142764848656952381134033203125;-0.067040192438827472809492746819159947335720062255859375;-0.028600678525859624112825940756010822951793670654296875;-0.452359910631902006894478063259157352149486541748046875;0.4009867174625458829950730432756245136260986328125;-0.239822770647339866822989051797776482999324798583984375;-0.470685619005303923501060126000083982944488525390625;-0.4068062304188486688616421815822832286357879638671875;0.9372201712705725551444402299239300191402435302734375;-0.99400142862411744459905094117857515811920166015625;-0.75301749780288673719041980803012847900390625;-0.234045308748025815415161332566640339791774749755859375;0.373406685408792071712014148943126201629638671875;-1.0597994395055365668412150625954382121562957763671875;0.314222984186316889321233247756026685237884521484375;-0.2078736406071655107297146969358436763286590576171875;-0.418901817343616700295427790479152463376522064208984375;-0.008801912503494602191267404123209416866302490234375;0.7107362770348044644919127676985226571559906005859375;0.7168103316080010056765559056657366454601287841796875]
      mask Display: e = 0.06;c1 = [120 150 230]/255;c2 = ([120 150 230]+0)/383;c3 = ([120 150 230]+128)/383;patch([0 1 1 0],[0 0 1 1],c1);patch([0 1 1 1-e 1-e 0+e],[0 0 1 1-e 0+e 0+e],c2);patch([0 0 1 1-e 0+e 0+e],[0 1 1 1-e 1-e 0+e],c3);plot([0 1 1 0 0],[0 0 1 1 0]);disp('weights');
  "IW{2,1}(5,:)'" : Constant  Value=[0.458385916159752326848320080898702144622802734375;0.84813204407613385082953527671634219586849212646484375;0.94650514098018889708185952258645556867122650146484375;0.74594759247516162492530611416441388428211212158203125;-0.104407762306979901012482514488510787487030029296875;0.1186644642958175899227768468335852958261966705322265625;1.1320098295769753793393874730099923908710479736328125;-0.179500407650915239088362795882858335971832275390625;0.771881138648502496124592653359286487102508544921875;-0.548635947097185994181245405343361198902130126953125;-0.6746199449777219303570063857478089630603790283203125;-0.360703913511002005609640264083282090723514556884765625;-0.597605875234097805304145367699675261974334716796875;-0.2568202039282214688142857994535006582736968994140625;0.5941759809159934402345015769242309033870697021484375;-0.039514724787864351218669156651230878196656703948974609375;0.229408580836399644820033927317126654088497161865234375;0.3342008973025247797750125755555927753448486328125;0.9800633193214773886126067736768163740634918212890625;0.5721963713908120308104798823478631675243377685546875]
      mask Display: e = 0.06;c1 = [120 150 230]/255;c2 = ([120 150 230]+0)/383;c3 = ([120 150 230]+128)/383;patch([0 1 1 0],[0 0 1 1],c1);patch([0 1 1 1-e 1-e 0+e],[0 0 1 1-e 0+e 0+e],c2);patch([0 0 1 1-e 0+e 0+e],[0 1 1 1-e 1-e 0+e],c3);plot([0 1 1 0 0],[0 0 1 1 0]);disp('weights');
  "IW{2,1}(6,:)'" : Constant  Value=[-0.77384781592172646735861007982748560607433319091796875;0.59108358077430744881297641768469475209712982177734375;-0.03728241009351639101421227451282902620732784271240234375;-0.97709174729592696007074437147821299731731414794921875;-0.7147538303215750232766367844305932521820068359375;-0.7829717176517638765886886176303960382938385009765625;-0.294662176883997595222552945415372960269451141357421875;-0.944338143760384607361402231617830693721771240234375;-0.17518116218259738303686390281654894351959228515625;0.51402311101222941669419697063858620822429656982421875;-0.99002176729454915982131524287979118525981903076171875;0.59043122934621827813117533878539688885211944580078125;-0.22370698215694329036296039703302085399627685546875;-1.056867006809679931933487750939093530178070068359375;0.4898055941529031453995912670507095754146575927734375;-0.6821680952663047303730081694084219634532928466796875;0.11879445532585231060096475630416534841060638427734375;-0.9976352361648259670090510553563944995403289794921875;-0.25460723909267901632347275153733789920806884765625;0.71721151247017311813891637939377687871456146240234375]
      mask Display: e = 0.06;c1 = [120 150 230]/255;c2 = ([120 150 230]+0)/383;c3 = ([120 150 230]+128)/383;patch([0 1 1 0],[0 0 1 1],c1);patch([0 1 1 1-e 1-e 0+e],[0 0 1 1-e 0+e 0+e],c2);patch([0 0 1 1-e 0+e 0+e],[0 1 1 1-e 1-e 0+e],c3);plot([0 1 1 0 0],[0 0 1 1 0]);disp('weights');
  "IW{2,1}(7,:)'" : Constant  Value=[-0.346106597572619578695451991734444163739681243896484375;0.399965489278604924283655464023468084633350372314453125;0.05447508061110746535593563066868227906525135040283203125;-0.87040339931752341851023402341525070369243621826171875;0.73883982147536653162234188130241818726062774658203125;0.427854113066676700061208293845993466675281524658203125;0.01403070065209728600752470129009452648460865020751953125;0.4861792379995455437580176294432021677494049072265625;0.9094214428940137207035832034307532012462615966796875;-0.03207414214986463452117249062212067656219005584716796875;-0.348223319994564739499054439875180833041667938232421875;0.269391913218515022254706536841695196926593780517578125;0.29729876555941192606269396492280066013336181640625;-0.3376447225389271888928988119005225598812103271484375;0.05065007115898811917986677144654095172882080078125;0.192316247203768775353438513775472529232501983642578125;0.02751917507898900272511610864967224188148975372314453125;0.54788988685930639643828499174560420215129852294921875;-0.0493641951991126148868715972639620304107666015625;-0.4195018892299196000550409735296852886676788330078125]
      mask Display: e = 0.06;c1 = [120 150 230]/255;c2 = ([120 150 230]+0)/383;c3 = ([120 150 230]+128)/383;patch([0 1 1 0],[0 0 1 1],c1);patch([0 1 1 1-e 1-e 0+e],[0 0 1 1-e 0+e 0+e],c2);patch([0 0 1 1-e 0+e 0+e],[0 1 1 1-e 1-e 0+e],c3);plot([0 1 1 0 0],[0 0 1 1 0]);disp('weights');
  "IW{2,1}(8,:)'" : Constant  Value=[-0.4222247145553748026713947183452546596527099609375;-0.21721956818752463647115291678346693515777587890625;-0.9040421881661249159378712647594511508941650390625;-0.3123401623225401380068433354608714580535888671875;-0.659182426027054901851442991755902767181396484375;0.1071026475764949026370231877081096172332763671875;0.284211002345112984102115660789422690868377685546875;0.632817971168942339232899030321277678012847900390625;-0.547292087681830796697113328264094889163970947265625;-0.3485709524739946107985133494366891682147979736328125;-0.41553914574393413516872897162102162837982177734375;0.24871299518162803821041961782611906528472900390625;0.1147721648015693762800992772099561989307403564453125;-0.7624419190360403053574600562569685280323028564453125;-0.4513177129819692101619921231758780777454376220703125;-0.6204052150719709946002922151819802820682525634765625;0.61410793186216050543180244858376681804656982421875;-0.5183224447713659088776694261468946933746337890625;-0.4326929827700409791901847711415030062198638916015625;-0.7244215935176316900623305627959780395030975341796875]
      mask Display: e = 0.06;c1 = [120 150 230]/255;c2 = ([120 150 230]+0)/383;c3 = ([120 150 230]+128)/383;patch([0 1 1 0],[0 0 1 1],c1);patch([0 1 1 1-e 1-e 0+e],[0 0 1 1-e 0+e 0+e],c2);patch([0 0 1 1-e 0+e 0+e],[0 1 1 1-e 1-e 0+e],c3);plot([0 1 1 0 0],[0 0 1 1 0]);disp('weights');
  "IW{2,1}(9,:)'" : Constant  Value=[-0.190978173858412481056490150876925326883792877197265625;-0.1996789391055066864577582919082487933337688446044921875;0.0179888509190704280749084631452205940149724483489990234375;0.327357546782829744724807596867321990430355072021484375;0.2104104813178007404861347140467842109501361846923828125;0.1477650701090928164749271900291205383837223052978515625;0.06591697331084343802753977570318966172635555267333984375;0.16383159435347227628199107130058109760284423828125;0.3252492492022092118730824950034730136394500732421875;-0.50858680198523220639117425889708101749420166015625;-0.428156892965022961572429949228535406291484832763671875;-0.387301045636488650014683798872283659875392913818359375;0.632655837397009701561501060496084392070770263671875;0.7909799836363540226358281870489008724689483642578125;0.7129675666138493017598420919966883957386016845703125;0.087806571408879985352058383796247653663158416748046875;-1.0488550692259883678758569658384658396244049072265625;0.83163734204239025959992659409181214869022369384765625;-0.1222137028141556669424971914850175380706787109375;0.7377144603656173860173339562606997787952423095703125]
      mask Display: e = 0.06;c1 = [120 150 230]/255;c2 = ([120 150 230]+0)/383;c3 = ([120 150 230]+128)/383;patch([0 1 1 0],[0 0 1 1],c1);patch([0 1 1 1-e 1-e 0+e],[0 0 1 1-e 0+e 0+e],c2);patch([0 0 1 1-e 0+e 0+e],[0 1 1 1-e 1-e 0+e],c3);plot([0 1 1 0 0],[0 0 1 1 0]);disp('weights');
  Mux : Mux  Inputs=20
      mask Display: e = 0.06;c1 = [120 150 230]/255;c2 = ([120 150 230]+0)/383;c3 = ([120 150 230]+128)/383;patch([0 1 1 0],[0 0 1 1],c1);patch([0 1 1 1-e 1-e 0+e],[0 0 1 1-e 0+e 0+e],c2);patch([0 0 1 1-e 0+e 0+e],[0 1 1 1-e 1-e 0+e],c3);plot([0 1 1 0 0],[0 0 1 1 0]);disp('Mux');
  dotprod{1..20} (20 alike) : neural/Weight Functions/dotprod
  "lz{2,1}" : Outport
      mask Display: e = 0.06;c1 = [120 230 180]/255;c2 = ([120 230 180]+0)/(256+128);c3 = ([120 230 180]+128)/(256+128);patch([0 1 1 0],[0 0 1 1],c1);patch([0 1 1 1-e 1-e 0+e],[0 0 1 1-e 0+e 0+e],c2);patch([0 0 1 1-e 0+e 0+e],[0 1 1 1-e 1-e 0+e],c3);plot([0 1 1 0 0],[0 0 1 1 0]);
  wires:
  "IW{2,1}(1,:)'"/1 -> dotprod1/1
  "ad{2,1}"/1 -> dotprod1/2, dotprod2/2, dotprod3/2, dotprod4/2, dotprod5/2, dotprod6/2, dotprod7/2, dotprod8/2, dotprod9/2, dotprod10/2, dotprod11/2, dotprod12/2, dotprod13/2, dotprod14/2, dotprod15/2, dotprod16/2, dotprod17/2, dotprod18/2, dotprod19/2, dotprod20/2
  dotprod1/1 -> Mux/1
  "IW{2,1}(2,:)'"/1 -> dotprod2/1
  dotprod2/1 -> Mux/2
  "IW{2,1}(3,:)'"/1 -> dotprod3/1
  dotprod3/1 -> Mux/3
  "IW{2,1}(4,:)'"/1 -> dotprod4/1
  dotprod4/1 -> Mux/4
  "IW{2,1}(5,:)'"/1 -> dotprod5/1
  dotprod5/1 -> Mux/5
  "IW{2,1}(6,:)'"/1 -> dotprod6/1
  dotprod6/1 -> Mux/6
  "IW{2,1}(7,:)'"/1 -> dotprod7/1
  dotprod7/1 -> Mux/7
  "IW{2,1}(8,:)'"/1 -> dotprod8/1
  dotprod8/1 -> Mux/8
  "IW{2,1}(9,:)'"/1 -> dotprod9/1
  dotprod9/1 -> Mux/9
  "IW{2,1}(10,:)'"/1 -> dotprod10/1
  dotprod10/1 -> Mux/10
  "IW{2,1}(11,:)'"/1 -> dotprod11/1
  dotprod11/1 -> Mux/11
  "IW{2,1}(12,:)'"/1 -> dotprod12/1
  dotprod12/1 -> Mux/12
  "IW{2,1}(13,:)'"/1 -> dotprod13/1
  dotprod13/1 -> Mux/13
  "IW{2,1}(14,:)'"/1 -> dotprod14/1
  dotprod14/1 -> Mux/14
  "IW{2,1}(15,:)'"/1 -> dotprod15/1
  dotprod15/1 -> Mux/15
  "IW{2,1}(16,:)'"/1 -> dotprod16/1
  dotprod16/1 -> Mux/16
  "IW{2,1}(17,:)'"/1 -> dotprod17/1
  dotprod17/1 -> Mux/17
  "IW{2,1}(18,:)'"/1 -> dotprod18/1
  dotprod18/1 -> Mux/18
  "IW{2,1}(19,:)'"/1 -> dotprod19/1
  dotprod19/1 -> Mux/19
  "IW{2,1}(20,:)'"/1 -> dotprod20/1
  dotprod20/1 -> Mux/20
  Mux/1 -> "lz{2,1}"/1

== system nn_fuel_control_4_20_1/Air Fuel Control Model 1/Feed-Forward Neural Network/Layer 3/Delays 1 ==
  "p{3}" : Inport  PortDimensions=20
      mask Display: e = 0.06;c1 = [120 230 180]/255;c2 = ([120 230 180]+0)/(256+128);c3 = ([120 230 180]+128)/(256+128);patch([0 1 1 0],[0 0 1 1],c1);patch([0 1 1 1-e 1-e 0+e],[0 0 1 1-e 0+e 0+e],c2);patch([0 0 1 1-e 0+e 0+e],[0 1 1 1-e 1-e 0+e],c3);plot([0 1 1 0 0],[0 0 1 1 0]);
  mux : Mux  Inputs=1
      mask Display: e = 0.06;c1 = [120 150 230]/255;c2 = ([120 150 230]+0)/383;c3 = ([120 150 230]+128)/383;patch([0 1 1 0],[0 0 1 1],c1);patch([0 1 1 1-e 1-e 0+e],[0 0 1 1-e 0+e 0+e],c2);patch([0 0 1 1-e 0+e 0+e],[0 1 1 1-e 1-e 0+e],c3);plot([0 1 1 0 0],[0 0 1 1 0]);disp('Mux')
  "pd{3,2}" : Outport
      mask Display: e = 0.06;c1 = [120 230 180]/255;c2 = ([120 230 180]+0)/(256+128);c3 = ([120 230 180]+128)/(256+128);patch([0 1 1 0],[0 0 1 1],c1);patch([0 1 1 1-e 1-e 0+e],[0 0 1 1-e 0+e 0+e],c2);patch([0 0 1 1-e 0+e 0+e],[0 1 1 1-e 1-e 0+e],c3);plot([0 1 1 0 0],[0 0 1 1 0]);
  wires:
  "p{3}"/1 -> mux/1
  mux/1 -> "pd{3,2}"/1
